simulink model "suspensionsignal"  (R2023b)
settings: Solver=ode15s  StartTime=0.0  StopTime=10.0  RelTol=1e-3
values from neighbouring files (symbols this model uses):
  c = 2    [main.m]
  k = 10    [main.m]
  total_mass = base_mass + load_mass    (= 40)    [main.m]
settings Model: Creator=franciscomigueljao  LastModifiedBy=kai

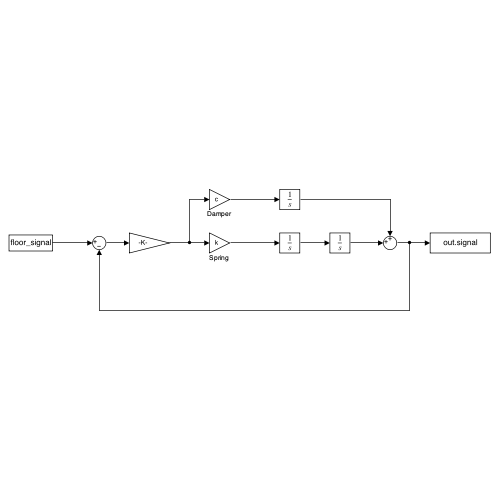
[thumbnail: Simulink's stored preview of the top-level diagram]
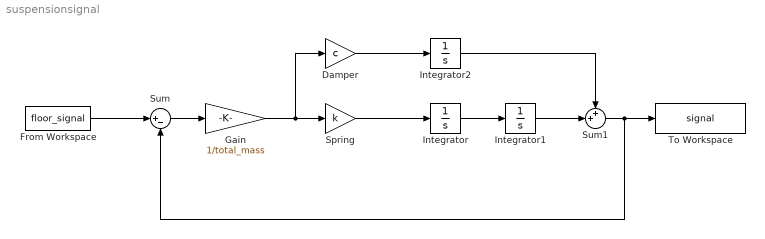
== system suspensionsignal ==
  Damper : Gain  Gain=c
  From Workspace : FromWorkspace  VariableName=floor_signal
  Gain : Gain  Gain=1/total_mass
  Integrator : Integrator
  Integrator1 : Integrator
  Integrator2 : Integrator
  Spring : Gain  Gain=k
  Sum : Sum  Inputs=|+-
  Sum1 : Sum  Inputs=++|
  To Workspace : ToWorkspace  VariableName=signal  SaveFormat=Timeseries  SampleTime=-1
  wires:
  Integrator/1 -> Integrator1/1
  Sum1/1 -> To Workspace/1, Sum/2
  From Workspace/1 -> Sum/1
  Sum/1 -> Gain/1
  Spring/1 -> Integrator/1
  Damper/1 -> Integrator2/1
  Integrator2/1 -> Sum1/1
  Integrator1/1 -> Sum1/2
  Gain/1 -> Damper/1, Spring/1
